simulink model "motor"  (R2022a)
settings: Solver=ode4  StartTime=0.0  StopTime=3  FixedStep=0.01  RelTol=1e-3
values from neighbouring files (symbols this model uses):
  b = 3.5077E-6    (= 3.5077e-06)    [params_setup.m]
  J = 3.2284E-6    (= 3.2284e-06)    [params_setup.m]
  Kb = 0.0274    [params_setup.m]
  Kt = 0.0274    [params_setup.m]
  L = 2.75E-6    (= 2.75e-06)    [params_setup.m]
  R = 4    [params_setup.m]
  V = 1    [params_setup.m]
settings Model: Creator=stakk  LastModifiedBy=stakk

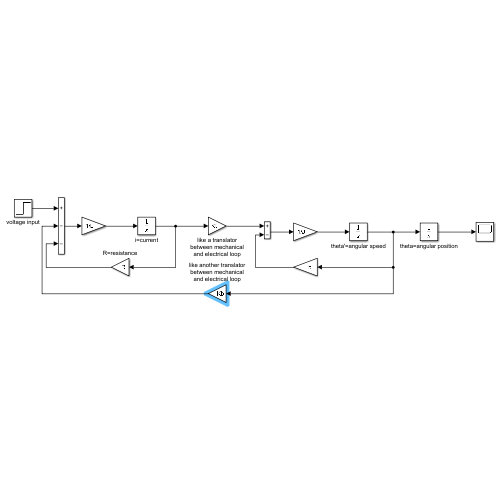
[thumbnail: Simulink's stored preview of the top-level diagram]
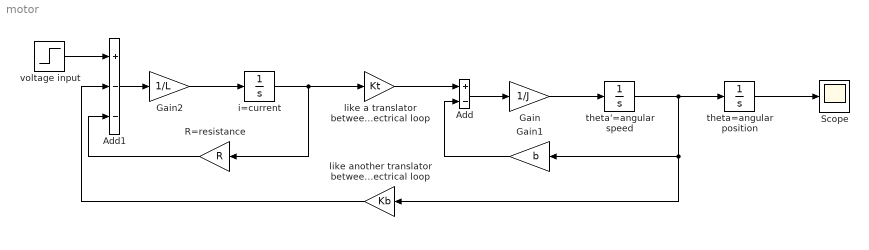
== system motor ==
  Add : Sum  Inputs=+-
  Add1 : Sum  Inputs=+--
  Gain : Gain  Gain=1/J
  Gain1 : Gain  Gain=b
  Gain2 : Gain  Gain=1/L
  R=resistance : Gain  Gain=R
  Scope : Scope
  i=current : Integrator
  like a translator between mechanical and electrical loop : Gain  Gain=Kt
  like another translator between mechanical and electrical loop : Gain  Gain=Kb
  theta'=angular speed : Integrator
  theta=angular position : Integrator
  voltage input : Step  After=V  SampleTime=0
  wires:
  theta'=angular speed/1 -> like another translator between mechanical and electrical loop/1, Gain1/1, theta=angular position/1
  Gain/1 -> theta'=angular speed/1
  Add/1 -> Gain/1
  Gain1/1 -> Add/2
  like a translator between mechanical and electrical loop/1 -> Add/1
  theta=angular position/1 -> Scope/1
  i=current/1 -> R=resistance/1, like a translator between mechanical and electrical loop/1
  Add1/1 -> Gain2/1
  voltage input/1 -> Add1/1
  R=resistance/1 -> Add1/3
  Gain2/1 -> i=current/1
  like another translator between mechanical and electrical loop/1 -> Add1/2
